simulink model "Yaw_simulink_pid"  (R2018b)
settings: Solver=VariableStepAuto  StartTime=0.0  StopTime=15  RelTol=1e-3
values from neighbouring files (symbols this model uses):
  beta = 63.4*pi/180    (= 1.10653874576)    [Spacecraft.m]
  int_resist = 50    [Spacecraft.m]
  Iw = max([Iw_roll Iw_pitch Iw_yaw])    [Spacecraft.m]    (also in maneuver.m = z2(end)*Is/(4*Omega_max*cos(beta)))
  Izz = 50000    [Spacecraft.m]
undefined symbols (not defined in the file or in its folder): N
libraries: cstblocks x2
settings Model: Creator=Lucie  LastModifiedBy=Lucie

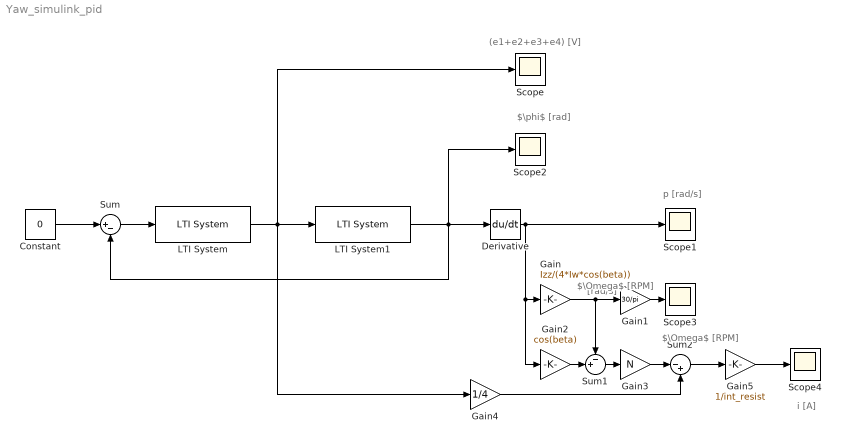
== system Yaw_simulink_pid ==
  note: i [A]
  note: [rad/s]
  note: $\Omega$ [RPM]
  note: $\phi$ [rad]
  note: (e1+e2+e3+e4) [V]
  note: p [rad/s]
  note: $\Omega$ [RPM]
  Constant : Constant  Value=0
  Derivative : Derivative
  Gain : Gain  Gain=Izz/(4*Iw*cos(beta))
  Gain1 : Gain  Gain=30/pi
  Gain2 : Gain  Gain=cos(beta)
  Gain3 : Gain  Gain=N
  Gain4 : Gain  Gain=1/4
  Gain5 : Gain  Gain=1/int_resist
  LTI System : cstblocks/LTI System  sys=C  IC=[]
  LTI System1 : cstblocks/LTI System  sys=Hy_pid  IC=[]
  Scope{,1..4} (5 alike) : Scope
  Sum : Sum  Inputs=|+-
  Sum1 : Sum  Inputs=-+|
  Sum2 : Sum  Inputs=|-+
  wires:
  LTI System/1 -> Gain4/1, LTI System1/1, Scope/1
  LTI System1/1 -> Derivative/1, Scope2/1, Sum/2
  Constant/1 -> Sum/1
  Sum/1 -> LTI System/1
  Derivative/1 -> Gain2/1, Gain/1, Scope1/1
  Gain/1 -> Sum1/1, Gain1/1
  Gain1/1 -> Scope3/1
  Gain2/1 -> Sum1/2
  Sum1/1 -> Gain3/1
  Gain3/1 -> Sum2/1
  Gain4/1 -> Sum2/2
  Sum2/1 -> Gain5/1
  Gain5/1 -> Scope4/1
